simulink model "IIR_filter_shell"  (R2020b)
settings: Solver=FixedStepDiscrete  StartTime=0.0  StopTime=10.0  RelTol=1e-3
model workspace (MATLAB code in the model file):
  | % VOICE BAND BANDPASS
  | 
  | fs = 48e3; %sampling frequency
  | flow = 0.2e3; Wlow = flow/(fs/2); %normalized flow
  | fhigh = 2.5e3; Whigh = fhigh/(fs/2); %normalized fhigh
  | n = 3; %filter order
  | PB_ripple = 1; %1db
  | SB_atten = 60; %60db attenuation
  | 
  | % Generate Elliptic IIR Filter Coefficients
  | [b,a] = ellip(n,PB_ripple,SB_atten,[Wlow Whigh], 'bandpass');
undefined symbols (not defined in the file or in its folder): a, b
settings Model: DataTypeOverride=Off  Creator=mcrisafu  LastModifiedBy=mcrisafu
settings OptimizationCC: BlockReduction=off  ConditionallyExecuteInputs=off  DefaultParameterBehavior=Inlined
settings DebuggingCC: AlgebraicLoopMsg=error  SingleTaskRateTransMsg=error
settings HardwareCC: ProdBitPerPointer=32  ProdBitPerSizeT=32  ProdBitPerPtrDiffT=32  ProdLargestAtomicFloat=None  ProdIntDivRoundTo=Undefined  ProdEndianess=Unspecified  ProdWordSize=32  ProdHWDeviceType=ASIC/FPGA->ASIC/FPGA  TargetBitPerLong=64  TargetBitPerPointer=64  TargetBitPerSizeT=64  TargetBitPerPtrDiffT=64  TargetLongLongMode=on  TargetIntDivRoundTo=Zero  TargetEndianess=LittleEndian  TargetWordSize=64  TargetHWDeviceType=Custom Processor->MATLAB Host Computer  ProdEqTarget=off

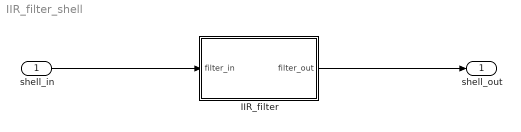
== system IIR_filter_shell ==
  shell_in : Inport
  IIR_filter : Subsystem
  shell_out : Outport  VectorParamsAs1DForOutWhenUnconnected=off
  wires:
  shell_in/1 -> IIR_filter/1(filter_in)
  IIR_filter/1(filter_out) -> shell_out/1

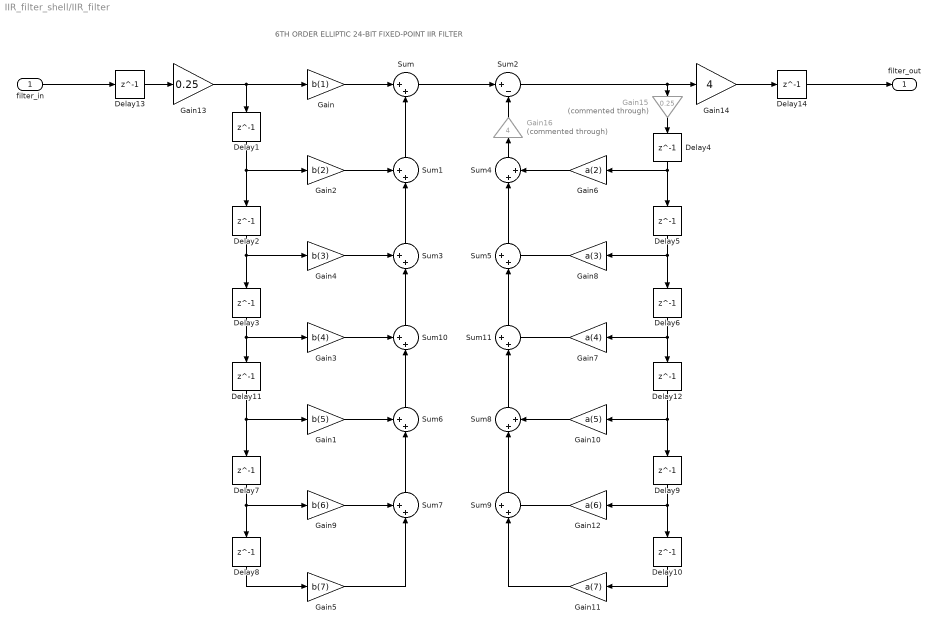
== system IIR_filter_shell/IIR_filter ==
  note: 6TH ORDER ELLIPTIC 24-BIT FIXED-POINT IIR FILTER
  filter_in : Inport  OutMin=[-1]  OutMax=[1]  OutDataTypeStr=fixdt(1,24)
  Delay{1..14} (14 alike) : Delay  DelayLength=1
  Gain : Gain  Gain=b(1)  OutMin=[-1]  OutMax=[1]  OutDataTypeStr=fixdt(1,24)
  Gain1 : Gain  Gain=b(5)  OutMin=[-1]  OutMax=[1]  OutDataTypeStr=fixdt(1,24)
  Gain10 : Gain  Gain=a(5)  OutMin=[-1]  OutMax=[1]  OutDataTypeStr=fixdt(1,24)
  Gain11 : Gain  Gain=a(7)  OutMin=[-1]  OutMax=[1]  OutDataTypeStr=fixdt(1,24)
  Gain12 : Gain  Gain=a(6)  OutMin=[-1]  OutMax=[1]  OutDataTypeStr=fixdt(1,24)
  Gain13 : Gain  Gain=0.25  OutMin=[-1]  OutMax=[1]  OutDataTypeStr=fixdt(1,24)
  Gain14 : Gain  Gain=4  OutMin=[-1]  OutMax=[1]  OutDataTypeStr=fixdt(1,24)
  Gain15 : Gain  Commented=through  Gain=0.25  OutMin=[-1]  OutMax=[1]  OutDataTypeStr=fixdt(1,24)
  Gain16 : Gain  Commented=through  Gain=4  OutMin=[-1]  OutMax=[1]  OutDataTypeStr=fixdt(1,24)
  Gain2 : Gain  Gain=b(2)  OutMin=[-1]  OutMax=[1]  OutDataTypeStr=fixdt(1,24)
  Gain3 : Gain  Gain=b(4)  OutMin=[-1]  OutMax=[1]  OutDataTypeStr=fixdt(1,24)
  Gain4 : Gain  Gain=b(3)  OutMin=[-1]  OutMax=[1]  OutDataTypeStr=fixdt(1,24)
  Gain5 : Gain  Gain=b(7)  OutMin=[-1]  OutMax=[1]  OutDataTypeStr=fixdt(1,24)
  Gain6 : Gain  Gain=a(2)  OutMin=[-1]  OutMax=[1]  OutDataTypeStr=fixdt(1,24)
  Gain7 : Gain  Gain=a(4)  OutMin=[-1]  OutMax=[1]  OutDataTypeStr=fixdt(1,24)
  Gain8 : Gain  Gain=a(3)  OutMin=[-1]  OutMax=[1]  OutDataTypeStr=fixdt(1,24)
  Gain9 : Gain  Gain=b(6)  OutMin=[-1]  OutMax=[1]  OutDataTypeStr=fixdt(1,24)
  Sum{,4..5,8..9,11} (6 alike) : Sum  Inputs=|++  OutMin=[-1]  OutMax=[1]  OutDataTypeStr=Inherit: Inherit via back propagation
  Sum{1,3,6..7,10} (5 alike) : Sum  Inputs=++|  OutMin=[-1]  OutMax=[1]  OutDataTypeStr=Inherit: Inherit via back propagation
  Sum2 : Sum  Inputs=|+-  OutMin=[-1]  OutMax=[1]  OutDataTypeStr=Inherit: Inherit via back propagation
  filter_out : Outport  OutMin=[-1]  OutMax=[1]  OutDataTypeStr=fixdt(1,24)
  wires:
  Gain/1 -> Sum/1
  Gain2/1 -> Sum1/1
  Sum1/1 -> Sum/2
  Delay1/1 -> Delay2/1, Gain2/1
  Gain4/1 -> Sum3/1
  Delay2/1 -> Delay3/1, Gain4/1
  Sum3/1 -> Sum1/2
  Delay3/1 -> Delay11/1, Gain3/1
  Delay6/1 -> Delay12/1, Gain7/1
  Delay5/1 -> Delay6/1, Gain8/1
  Delay4/1 -> Delay5/1, Gain6/1
  Gain6/1 -> Sum4/2
  Gain8/1 -> Sum5/2
  Sum5/1 -> Sum4/1
  Sum/1 -> Sum2/1
  Sum4/1 -> Gain16/1
  Sum9/1 -> Sum8/1
  Delay11/1 -> Delay7/1, Gain1/1
  Gain9/1 -> Sum7/1
  Sum7/1 -> Sum6/2
  Gain12/1 -> Sum9/2
  Delay7/1 -> Delay8/1, Gain9/1
  Gain10/1 -> Sum8/2
  Delay10/1 -> Gain11/1
  Delay12/1 -> Delay9/1, Gain10/1
  Delay8/1 -> Gain5/1
  Gain1/1 -> Sum6/1
  Sum6/1 -> Sum10/2
  Sum8/1 -> Sum11/1
  Delay9/1 -> Delay10/1, Gain12/1
  Sum11/1 -> Sum5/1
  Sum10/1 -> Sum3/2
  Gain3/1 -> Sum10/1
  Gain7/1 -> Sum11/2
  Gain5/1 -> Sum7/2
  Gain11/1 -> Sum9/1
  filter_in/1 -> Delay13/1
  Sum2/1 -> Gain14/1, Gain15/1
  Delay13/1 -> Gain13/1
  Delay14/1 -> filter_out/1
  Gain13/1 -> Delay1/1, Gain/1
  Gain14/1 -> Delay14/1
  Gain15/1 -> Delay4/1
  Gain16/1 -> Sum2/2
